simulink model "b_tau_model"  (R2023b)
settings: Solver=VariableStepAuto  StartTime=0.0  StopTime=10.0  RelTol=1e-3
values from neighbouring files (symbols this model uses):
  k_i = constantes(15)    [calculaMatrizesModelo.m]    (also in simulaModeloSimulink.m; simulaTrajetoriaSimulink.m)
  k_p = constantes(16)    [calculaMatrizesModelo.m]    (also in simulaModeloSimulink.m; simulaTrajetoriaSimulink.m)
  K_t = constantes(9)    [calculaMatrizesModelo.m]    (also in simulaModeloSimulink.m; simulaTrajetoriaSimulink.m)
  R_a = constantes(10)    [calculaMatrizesModelo.m]    (also in simulaModeloSimulink.m; simulaTrajetoriaSimulink.m)
settings Model: Creator=Gabriel Sousa  LastModifiedBy=Gabriel Sousa

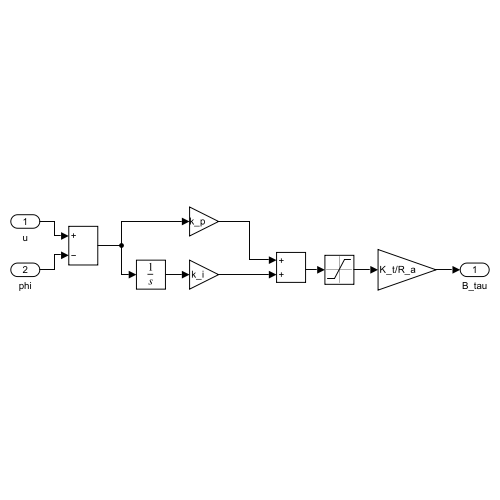
[thumbnail: Simulink's stored preview of the top-level diagram]
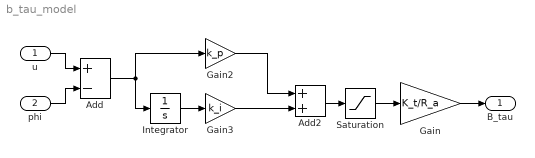
== system b_tau_model ==
  u : Inport
  phi : Inport  Port=2
  Add : Sum  Inputs=+-
  Add2 : Sum
  Gain : Gain  Gain=K_t/R_a
  Gain2 : Gain  Gain=k_p
  Gain3 : Gain  Gain=k_i
  Integrator : Integrator
  Saturation : Saturate  UpperLimit=12  LowerLimit=-12
  B_tau : Outport
  wires:
  Integrator/1 -> Gain3/1
  Add/1 -> Gain2/1, Integrator/1
  Gain3/1 -> Add2/2
  u/1 -> Add/1
  Gain2/1 -> Add2/1
  phi/1 -> Add/2
  Gain/1 -> B_tau/1
  Add2/1 -> Saturation/1
  Saturation/1 -> Gain/1
